simulink model "double_3D_pend"  (R2023a)
settings: Solver=VariableStepAuto  StartTime=0.0  StopTime=5  MaxStep=1e-3  RelTol=1e-9  AbsTol=1e-9  EnableMultiTasking=on
InitFcn:
  | addpath quaternion_muscle\
  | data;
values from neighbouring files (symbols this model uses):
  akt = [1,1,1]    [data.m]    (also in odvozeni_svaly.m = sym('akt',[1 6]); optim_control_nlmpc.m = u'; simulation.m = [1,1,1]*0.5)
  c = 0    [data.m]    (also in neco.m = cos(0); optim_control_nlmpc.m = 100; simulation.m = 10)
  force = [1,1,0]*(-30)    [data.m]    (also in odvozeni_svaly.m = (((length / l0m)^3) * exp(8 * length / l0m - 12.9) + (exp(-(; optim_control_nlmpc.m = [1,1,1,1,1,1]*(30); simulation.m = -[1,2,1]*1)
  g = 9.81    [data.m]    (also in optim_control_nlmpc.m; simulation.m)
  IL = [8.1667, 8.1667, 1.66667,0,0,0]    [data.m]    (also in fo_python_to_matlab.m = [ILxx ILyy ILzz ILxy ILyz ILzx]; mm_python_to_matlab.m = [ILxx ILyy ILzz ILxy ILyz ILzx]; optim_control_nlmpc.m; simulation.m = [84.1667, 84.1667, 1.66667])
  initialConditions = [1,0,0,0,0,0,zeros(1,6)]*2    [data.m]    (also in simulation.m = [1,1,1,1,1,1,0,0,0,0,0,0]*0)
  IU = [8.1667, 8.1667, 1.66667,0,0,0]    [data.m]    (also in fo_python_to_matlab.m = [IUxx IUyy IUzz IUxy IUyz IUzx]; mm_python_to_matlab.m = [IUxx IUyy IUzz IUxy IUyz IUzx]; optim_control_nlmpc.m; simulation.m = [84.1667, 84.1667, 1.66667]*1e-2)
  k = 100    [data.m]    (also in neco.m = elips_pars.k; optim_control_nlmpc.m = 0; simulation.m = 1)
  l0m = [12,25,15]    [data.m]    (also in odvozeni_svaly.m = sym('l0m', [1 6]); optim_control_nlmpc.m = [30,30,30,30,30,30]; simulation.m = [10,20,10])
  m = rand(1,2)*10    [data.m]    (also in fo_python_to_matlab.m = [m1,m2]; mm_python_to_matlab.m = [m1,m2]; neco.m = elips_pars.m; optim_control_nlmpc.m = [5,10])
  rigid1C = [0,0,5]    [data.m]    (also in fo_python_to_matlab.m = [rigid1Cx, rigid1Cy, rigid1Cz]; mm_python_to_matlab.m = [rigid1Cx, rigid1Cy, rigid1Cz]; optim_control_nlmpc.m)
  rigid1P = [0,0,-5]    [data.m]    (also in fo_python_to_matlab.m = [rigid1Px, rigid1Py, rigid1Pz]; mm_python_to_matlab.m = [rigid1Px, rigid1Py, rigid1Pz]; optim_control_nlmpc.m)
  rigid2C = [0,0,5]    [data.m]    (also in fo_python_to_matlab.m = [rigid2Cx, rigid2Cy, rigid2Cz]; mm_python_to_matlab.m = [rigid2Cx, rigid2Cy, rigid2Cz]; optim_control_nlmpc.m)
  s = sin(0)    [neco.m]
undefined symbols (not defined in the file or in its folder): Ixx, Iyy, Izz, l, q1init, q2init, X, Y, Z
libraries: sm_lib x104, nesl_utility x52
(part 5 of 5)

== matlab function double_3D_pend/MATLAB Function2 ==
  data: R output; pos1 input; vel1 input; acc1 input; pos2 input; vel2 input; acc2 input; g input
function R = fcn(pos1,vel1,acc1,pos2,vel2,acc2,g)
m1 = 5;
m2 = 10;

rigid1Cx = 0;
rigid1Cy = 0;
rigid1Cz = 5;

rigid1Px = 0;
rigid1Py = 0;
rigid1Pz = -5;

rigid2Cx = 0;
rigid2Cy = 0;
rigid2Cz = 5;

x1 = pos1(1);
x2 = pos1(2);
x3 = pos1(3);

dx1 = vel1(1);
dx2 = vel1(2);
dx3 = vel1(3);

ddx1 = acc1(1);
ddx2 = acc1(2);
ddx3 = acc1(3);

x4 = pos2(1);
x5 = pos2(2);
x6 = pos2(3);

dx4 = vel2(1);
dx5 = vel2(2);
dx6 = vel2(3);

ddx4 = acc2(1);
ddx5 = acc2(2);
ddx6 = acc2(3);

R = [m2.*((sin(x4).*sin(x6) - sin(x5).*cos(x4).*cos(x6)).*sin(x2) - (sin(x4).*sin(x5).*cos(x6) + sin(x6).*cos(x4)).*sin(x3).*cos(x2) + cos(x2).*cos(x3).*cos(x5).*cos(x6)).*(rigid2Cy.*(ddx4.*sin(x5) + ddx6 + dx4.*dx5.*cos(x5) - dx4.*(dx1.*sin(x2) + dx3).*sin(x4).*cos(x5) - dx4.*(-dx1.*sin(x3).*cos(x2) + dx2.*cos(x3)).*cos(x4).*cos(x5) - dx5.*(dx1.*sin(x2) + dx3).*sin(x5).*cos(x4) + dx5.*(-dx1.*sin(x3).*cos(x2) + dx2.*cos(x3)).*sin(x4).*sin(x5) + dx5.*(dx1.*cos(x2).*cos(x3) + dx2.*sin(x3)).*cos(x5) + (ddx1.*sin(x2) + ddx3 + dx1.*dx2.*cos(x2)).*cos(x4).*cos(x5) - (-ddx1.*sin(x3).*cos(x2) + ddx2.*cos(x3) + dx1.*dx2.*sin(x2).*sin(x3) - dx1.*dx3.*cos(x2).*cos(x3) - dx2.*dx3.*sin(x3)).*sin(x4).*cos(x5) + (ddx1.*cos(x2).*cos(x3) + ddx2.*sin(x3) - dx1.*dx2.*sin(x2).*cos(x3) - dx1.*dx3.*sin(x3).*cos(x2) + dx2.*dx3.*cos(x3)).*sin(x5)) - rigid2Cz.*(-ddx4.*sin(x6).*cos(x5) + ddx5.*cos(x6) + dx4.*dx5.*sin(x5).*sin(x6) - dx4.*dx6.*cos(x5).*cos(x6) - dx5.*dx6.*sin(x6) + dx5.*(dx1.*cos(x2).*cos(x3) + dx2.*sin(x3)).*sin(x5).*sin(x6) - dx6.*(dx1.*cos(x2).*cos(x3) + dx2.*sin(x3)).*cos(x5).*cos(x6) + (dx1.*sin(x2) + dx3).*(-dx4.*sin(x4).*sin(x5).*sin(x6) + dx4.*cos(x4).*cos(x6) + dx5.*sin(x6).*cos(x4).*cos(x5) - dx6.*sin(x4).*sin(x6) + dx6.*sin(x5).*cos(x4).*cos(x6)) + (sin(x4).*cos(x6) + sin(x5).*sin(x6).*cos(x4)).*(ddx1.*sin(x2) + ddx3 + dx1.*dx2.*cos(x2)) + (-dx1.*sin(x3).*cos(x2) + dx2.*cos(x3)).*(-dx4.*sin(x4).*cos(x6) - dx4.*sin(x5).*sin(x6).*cos(x4) - dx5.*sin(x4).*sin(x6).*cos(x5) - dx6.*sin(x4).*sin(x5).*cos(x6) - dx6.*sin(x6).*cos(x4)) + (-sin(x4).*sin(x5).*sin(x6) + cos(x4).*cos(x6)).*(-ddx1.*sin(x3).*cos(x2) + ddx2.*cos(x3) + dx1.*dx2.*sin(x2).*sin(x3) - dx1.*dx3.*cos(x2).*cos(x3) - dx2.*dx3.*sin(x3)) - (ddx1.*cos(x2).*cos(x3) + ddx2.*sin(x3) - dx1.*dx2.*sin(x2).*cos(x3) - dx1.*dx3.*sin(x3).*cos(x2) + dx2.*dx3.*cos(x3)).*sin(x6).*cos(x5)) - (-rigid2Cx.*(dx4.*sin(x5) + dx6 + (dx1.*sin(x2) + dx3).*cos(x4).*cos(x5) - (-dx1.*sin(x3).*cos(x2) + dx2.*cos(x3)).*sin(x4).*cos(x5) + (dx1.*cos(x2).*cos(x3) + dx2.*sin(x3)).*sin(x5)) + rigid2Cz.*(dx4.*cos(x5).*cos(x6) + dx5.*sin(x6) + (dx1.*sin(x2) + dx3).*(sin(x4).*sin(x6) - sin(x5).*cos(x4).*cos(x6)) + (-dx1.*sin(x3).*cos(x2) + dx2.*cos(x3)).*(sin(x4).*sin(x5).*cos(x6) + sin(x6).*cos(x4)) + (dx1.*cos(x2).*cos(x3) + dx2.*sin(x3)).*cos(x5).*cos(x6))).*(dx4.*sin(x5) + dx6 + (dx1.*sin(x2) + dx3).*cos(x4).*cos(x5) - (-dx1.*sin(x3).*cos(x2) + dx2.*cos(x3)).*sin(x4).*cos(x5) + (dx1.*cos(x2).*cos(x3) + dx2.*sin(x3)).*sin(x5)) + (rigid2Cx.*(-dx4.*sin(x6).*cos(x5) + dx5.*cos(x6) + (dx1.*sin(x2) + dx3).*(sin(x4).*cos(x6) + sin(x5).*sin(x6).*cos(x4)) + (-dx1.*sin(x3).*cos(x2) + dx2.*cos(x3)).*(-sin(x4).*sin(x5).*sin(x6) + cos(x4).*cos(x6)) - (dx1.*cos(x2).*cos(x3) + dx2.*sin(x3)).*sin(x6).*cos(x5)) - rigid2Cy.*(dx4.*cos(x5).*cos(x6) + dx5.*sin(x6) + (dx1.*sin(x2) + dx3).*(sin(x4).*sin(x6) - sin(x5).*cos(x4).*cos(x6)) + (-dx1.*sin(x3).*cos(x2) + dx2.*cos(x3)).*(sin(x4).*sin(x5).*cos(x6) + sin(x6).*cos(x4)) + (dx1.*cos(x2).*cos(x3) + dx2.*sin(x3)).*cos(x5).*cos(x6))).*(-dx4.*sin(x6).*cos(x5) + dx5.*cos(x6) + (dx1.*sin(x2) + dx3).*(sin(x4).*cos(x6) + sin(x5).*sin(x6).*cos(x4)) + (-dx1.*sin(x3).*cos(x2) + dx2.*cos(x3)).*(-sin(x4).*sin(x5).*sin(x6) + cos(x4).*cos(x6)) - (dx1.*cos(x2).*cos(x3) + dx2.*sin(x3)).*sin(x6).*cos(x5))) + m2.*((sin(x4).*cos(x6) + sin(x5).*sin(x6).*cos(x4)).*sin(x2) - (-sin(x4).*sin(x5).*sin(x6) + cos(x4).*cos(x6)).*sin(x3).*cos(x2) - sin(x6).*cos(x2).*cos(x3).*cos(x5)).*(-rigid2Cx.*(ddx4.*sin(x5) + ddx6 + dx4.*dx5.*cos(x5) - dx4.*(dx1.*sin(x2) + dx3).*sin(x4).*cos(x5) - dx4.*(-dx1.*sin(x3).*cos(x2) + dx2.*cos(x3)).*cos(x4).*cos(x5) - dx5.*(dx1.*sin(x2) + dx3).*sin(x5).*cos(x4) + dx5.*(-dx1.*sin(x3).*cos(x2) + dx2.*cos(x3)).*sin(x4).*sin(x5) + dx5.*(dx1.*cos(x2).*cos(x3) + dx2.*sin(x3)).*cos(x5) + (ddx1.*sin(x2) + ddx3 + dx1.*dx2.*cos(x2)).*cos(x4).*cos(x5) - (-ddx1.*sin(x3).*cos(x2) + ddx2.*cos(x3) + dx1.*dx2.*sin(x2).*sin(x3) - dx1.*dx3.*cos(x2).*cos(x3) - dx2.*dx3.*sin(x3)).*sin(x4).*cos(x5) + (ddx1.*cos(x2).*cos(x3) + ddx2.*sin(x3) - dx1.*dx2.*sin(x2).*cos(x3) - dx1.*dx3.*sin(x3).*cos(x2) + dx2.*dx3.*cos(x3)).*sin(x5)) + rigid2Cz.*(ddx4.*cos(x5).*cos(x6) + ddx5.*sin(x6) - dx4.*dx5.*sin(x5).*cos(x6) - dx4.*dx6.*sin(x6).*cos(x5) + dx5.*dx6.*cos(x6) - dx5.*(dx1.*cos(x2).*cos(x3) + dx2.*sin(x3)).*sin(x5).*cos(x6) - dx6.*(dx1.*cos(x2).*cos(x3) + dx2.*sin(x3)).*sin(x6).*cos(x5) + (dx1.*sin(x2) + dx3).*(dx4.*sin(x4).*sin(x5).*cos(x6) + dx4.*sin(x6).*cos(x4) - dx5.*cos(x4).*cos(x5).*cos(x6) + dx6.*sin(x4).*cos(x6) + dx6.*sin(x5).*sin(x6).*cos(x4)) + (sin(x4).*sin(x6) - sin(x5).*cos(x4).*cos(x6)).*(ddx1.*sin(x2) + ddx3 + dx1.*dx2.*cos(x2)) + (-dx1.*sin(x3).*cos(x2) + dx2.*cos(x3)).*(-dx4.*sin(x4).*sin(x6) + dx4.*sin(x5).*cos(x4).*cos(x6) + dx5.*sin(x4).*cos(x5).*cos(x6) - dx6.*sin(x4).*sin(x5).*sin(x6) + dx6.*cos(x4).*cos(x6)) + (sin(x4).*sin(x5).*cos(x6) + sin(x6).*cos(x4)).*(-ddx1.*sin(x3).*cos(x2) + ddx2.*cos(x3) + dx1.*dx2.*sin(x2).*sin(x3) - dx1.*dx3.*cos(x2).*cos(x3) - dx2.*dx3.*sin(x3)) + (ddx1.*cos(x2).*cos(x3) + ddx2.*sin(x3) - dx1.*dx2.*sin(x2).*cos(x3) - dx1.*dx3.*sin(x3).*cos(x2) + dx2.*dx3.*cos(x3)).*cos(x5).*cos(x6)) - (rigid2Cx.*(-dx4.*sin(x6).*cos(x5) + dx5.*cos(x6) + (dx1.*sin(x2) + dx3).*(sin(x4).*cos(x6) + sin(x5).*sin(x6).*cos(x4)) + (-dx1.*sin(x3).*cos(x2) + dx2.*cos(x3)).*(-sin(x4).*sin(x5).*sin(x6) + cos(x4).*cos(x6)) - (dx1.*cos(x2).*cos(x3) + dx2.*sin(x3)).*sin(x6).*cos(x5)) - rigid2Cy.*(dx4.*cos(x5).*cos(x6) + dx5.*sin(x6) + (dx1.*sin(x2) + dx3).*(sin(x4).*sin(x6) - sin(x5).*cos(x4).*cos(x6)) + (-dx1.*sin(x3).*cos(x2) + dx2.*cos(x3)).*(sin(x4).*sin(x5).*cos(x6) + sin(x6).*cos(x4)) + (dx1.*cos(x2).*cos(x3) + dx2.*sin(x3)).*cos(x5).*cos(x6))).*(dx4.*cos(x5).*cos(x6) + dx5.*sin(x6) + (dx1.*sin(x2) + dx3).*(sin(x4).*sin(x6) - sin(x5).*cos(x4).*cos(x6)) + (-dx1.*sin(x3).*cos(x2) + dx2.*cos(x3)).*(sin(x4).*sin(x5).*cos(x6) + sin(x6).*cos(x4)) + (dx1.*cos(x2).*cos(x3) + dx2.*sin(x3)).*cos(x5).*cos(x6)) + (rigid2Cy.*(dx4.*sin(x5) + dx6 + (dx1.*sin(x2) + dx3).*cos(x4).*cos(x5) - (-dx1.*sin(x3).*cos(x2) + dx2.*cos(x3)).*sin(x4).*cos(x5) + (dx1.*cos(x2).*cos(x3) + dx2.*sin(x3)).*sin(x5)) - rigid2Cz.*(-dx4.*sin(x6).*cos(x5) + dx5.*cos(x6) + (dx1.*sin(x2) + dx3).*(sin(x4).*cos(x6) + sin(x5).*sin(x6).*cos(x4)) + (-dx1.*sin(x3).*cos(x2) + dx2.*cos(x3)).*(-sin(x4).*sin(x5).*sin(x6) + cos(x4).*cos(x6)) - (dx1.*cos(x2).*cos(x3) + dx2.*sin(x3)).*sin(x6).*cos(x5))).*(dx4.*sin(x5) + dx6 + (dx1.*sin(x2) + dx3).*cos(x4).*cos(x5) - (-dx1.*sin(x3).*cos(x2) + dx2.*cos(x3)).*sin(x4).*cos(x5) + (dx1.*cos(x2).*cos(x3) + dx2.*sin(x3)).*sin(x5))) + m2.*(sin(x2).*cos(x4).*cos(x5) + sin(x3).*sin(x4).*cos(x2).*cos(x5) + sin(x5).*cos(x2).*cos(x3)).*(rigid2Cx.*(-ddx4.*sin(x6).*cos(x5) + ddx5.*cos(x6) + dx4.*dx5.*sin(x5).*sin(x6) - dx4.*dx6.*cos(x5).*cos(x6) - dx5.*dx6.*sin(x6) + dx5.*(dx1.*cos(x2).*cos(x3) + dx2.*sin(x3)).*sin(x5).*sin(x6) - dx6.*(dx1.*cos(x2).*cos(x3) + dx2.*sin(x3)).*cos(x5).*cos(x6) + (dx1.*sin(x2) + dx3).*(-dx4.*sin(x4).*sin(x5).*sin(x6) + dx4.*cos(x4).*cos(x6) + dx5.*sin(x6).*cos(x4).*cos(x5) - dx6.*sin(x4).*sin(x6) + dx6.*sin(x5).*cos(x4).*cos(x6)) + (sin(x4).*cos(x6) + sin(x5).*sin(x6).*cos(x4)).*(ddx1.*sin(x2) + ddx3 + dx1.*dx2.*cos(x2)) + (-dx1.*sin(x3).*cos(x2) + dx2.*cos(x3)).*(-dx4.*sin(x4).*cos(x6) - dx4.*sin(x5).*sin(x6).*cos(x4) - dx5.*sin(x4).*sin(x6).*cos(x5) - dx6.*sin(x4).*sin(x5).*cos(x6) - dx6.*sin(x6).*cos(x4)) + (-sin(x4).*sin(x5).*sin(x6) + cos(x4).*cos(x6)).*(-ddx1.*sin(x3).*cos(x2) + ddx2.*cos(x3) + dx1.*dx2.*sin(x2).*sin(x3) - dx1.*dx3.*cos(x2).*cos(x3) - dx2.*dx3.*sin(x3)) - (ddx1.*cos(x2).*cos(x3) + ddx2.*sin(x3) - dx1.*dx2.*sin(x2).*cos(x3) - dx1.*dx3.*sin(x3).*cos(x2) + dx2.*dx3.*cos(x3)).*sin(x6).*cos(x5)) - rigid2Cy.*(ddx4.*cos(x5).*cos(x6) + ddx5.*sin(x6) - dx4.*dx5.*sin(x5).*cos(x6) - dx4.*dx6.*sin(x6).*cos(x5) + dx5.*dx6.*cos(x6) - dx5.*(dx1.*cos(x2).*cos(x3) + dx2.*sin(x3)).*sin(x5).*cos(x6) - dx6.*(dx1.*cos(x2).*cos(x3) + dx2.*sin(x3)).*sin(x6).*cos(x5) + (dx1.*sin(x2) + dx3).*(dx4.*sin(x4).*sin(x5).*cos(x6) + dx4.*sin(x6).*cos(x4) - dx5.*cos(x4).*cos(x5).*cos(x6) + dx6.*sin(x4).*cos(x6) + dx6.*sin(x5).*sin(x6).*cos(x4)) + (sin(x4).*sin(x6) - sin(x5).*cos(x4).*cos(x6)).*(ddx1.*sin(x2) + ddx3 + dx1.*dx2.*cos(x2)) + (-dx1.*sin(x3).*cos(x2) + dx2.*cos(x3)).*(-dx4.*sin(x4).*sin(x6) + dx4.*sin(x5).*cos(x4).*cos(x6) + dx5.*sin(x4).*cos(x5).*cos(x6) - dx6.*sin(x4).*sin(x5).*sin(x6) + dx6.*cos(x4).*cos(x6)) + (sin(x4).*sin(x5).*cos(x6) + sin(x6).*cos(x4)).*(-ddx1.*sin(x3).*cos(x2) + ddx2.*cos(x3) + dx1.*dx2.*sin(x2).*sin(x3) - dx1.*dx3.*cos(x2).*cos(x3) - dx2.*dx3.*sin(x3)) + (ddx1.*cos(x2).*cos(x3) + ddx2.*sin(x3) - dx1.*dx2.*sin(x2).*cos(x3) - dx1.*dx3.*sin(x3).*cos(x2) + dx2.*dx3.*cos(x3)).*cos(x5).*cos(x6)) + (-rigid2Cx.*(dx4.*sin(x5) + dx6 + (dx1.*sin(x2) + dx3).*cos(x4).*cos(x5) - (-dx1.*sin(x3).*cos(x2) + dx2.*cos(x3)).*sin(x4).*cos(x5) + (dx1.*cos(x2).*cos(x3) + dx2.*sin(x3)).*sin(x5)) + rigid2Cz.*(dx4.*cos(x5).*cos(x6) + dx5.*sin(x6) + (dx1.*sin(x2) + dx3).*(sin(x4).*sin(x6) - sin(x5).*cos(x4).*cos(x6)) + (-dx1.*sin(x3).*cos(x2) + dx2.*cos(x3)).*(sin(x4).*sin(x5).*cos(x6) + sin(x6).*cos(x4)) + (dx1.*cos(x2).*cos(x3) + dx2.*sin(x3)).*cos(x5).*cos(x6))).*(dx4.*cos(x5).*cos(x6) + dx5.*sin(x6) + (dx1.*sin(x2) + dx3).*(sin(x4).*sin(x6) - sin(x5).*cos(x4).*cos(x6)) + (-dx1.*sin(x3).*cos(x2) + dx2.*cos(x3)).*(sin(x4).*sin(x5).*cos(x6) + sin(x6).*cos(x4)) + (dx1.*cos(x2).*cos(x3) + dx2.*sin(x3)).*cos(x5).*cos(x6)) - (rigid2Cy.*(dx4.*sin(x5) + dx6 + (dx1.*sin(x2) + dx3).*cos(x4).*cos(x5) - (-dx1.*sin(x3).*cos(x2) + dx2.*cos(x3)).*sin(x4).*cos(x5) + (dx1.*cos(x2).*cos(x3) + dx2.*sin(x3)).*sin(x5)) - rigid2Cz.*(-dx4.*sin(x6).*cos(x5) + dx5.*cos(x6) + (dx1.*sin(x2) + dx3).*(sin(x4).*cos(x6) + sin(x5).*sin(x6).*cos(x4)) + (-dx1.*sin(x3).*cos(x2) + dx2.*cos(x3)).*(-sin(x4).*sin(x5).*sin(x6) + cos(x4).*cos(x6)) - (dx1.*cos(x2).*cos(x3) + dx2.*sin(x3)).*sin(x6).*cos(x5))).*(-dx4.*sin(x6).*cos(x5) + dx5.*cos(x6) + (dx1.*sin(x2) + dx3).*(sin(x4).*cos(x6) + sin(x5).*sin(x6).*cos(x4)) + (-dx1.*sin(x3).*cos(x2) + dx2.*cos(x3)).*(-sin(x4).*sin(x5).*sin(x6) + cos(x4).*cos(x6)) - (dx1.*cos(x2).*cos(x3) + dx2.*sin(x3)).*sin(x6).*cos(x5))) - (m1.*(-rigid1Cx.*(ddx1.*sin(x2) + ddx3 + dx1.*dx2.*cos(x2)) + rigid1Cz.*(ddx1.*cos(x2).*cos(x3) + ddx2.*sin(x3) - dx1.*dx2.*sin(x2).*cos(x3) - dx1.*dx3.*sin(x3).*cos(x2) + dx2.*dx3.*cos(x3)) + (dx1.*sin(x2) + dx3).*(rigid1Cy.*(dx1.*sin(x2) + dx3) - rigid1Cz.*(-dx1.*sin(x3).*cos(x2) + dx2.*cos(x3))) - (rigid1Cx.*(-dx1.*sin(x3).*cos(x2) + dx2.*cos(x3)) - rigid1Cy.*(dx1.*cos(x2).*cos(x3) + dx2.*sin(x3))).*(dx1.*cos(x2).*cos(x3) + dx2.*sin(x3))) + m2.*(-rigid1Cx.*(ddx1.*sin(x2) + ddx3 + dx1.*dx2.*cos(x2)) + rigid1Cz.*(ddx1.*cos(x2).*cos(x3) + ddx2.*sin(x3) - dx1.*dx2.*sin(x2).*cos(x3) - dx1.*dx3.*sin(x3).*cos(x2) + dx2.*dx3.*cos(x3)) + rigid1Px.*(ddx1.*sin(x2) + ddx3 + dx1.*dx2.*cos(x2)) - rigid1Pz.*(ddx1.*cos(x2).*cos(x3) + ddx2.*sin(x3) - dx1.*dx2.*sin(x2).*cos(x3) - dx1.*dx3.*sin(x3).*cos(x2) + dx2.*dx3.*cos(x3)) + (dx1.*sin(x2) + dx3).*(rigid1Cy.*(dx1.*sin(x2) + dx3) - rigid1Cz.*(-dx1.*sin(x3).*cos(x2) + dx2.*cos(x3)) - rigid1Py.*(dx1.*sin(x2) + dx3) + rigid1Pz.*(-dx1.*sin(x3).*cos(x2) + dx2.*cos(x3))) - (dx1.*cos(x2).*cos(x3) + dx2.*sin(x3)).*(rigid1Cx.*(-dx1.*sin(x3).*cos(x2) + dx2.*cos(x3)) - rigid1Cy.*(dx1.*cos(x2).*cos(x3) + dx2.*sin(x3)) - rigid1Px.*(-dx1.*sin(x3).*cos(x2) + dx2.*cos(x3)) + rigid1Py.*(dx1.*cos(x2).*cos(x3) + dx2.*sin(x3))))).*sin(x3).*cos(x2) + (m1.*(rigid1Cx.*(-ddx1.*sin(x3).*cos(x2) + ddx2.*cos(x3) + dx1.*dx2.*sin(x2).*sin(x3) - dx1.*dx3.*cos(x2).*cos(x3) - dx2.*dx3.*sin(x3)) - rigid1Cy.*(ddx1.*cos(x2).*cos(x3) + ddx2.*sin(x3) - dx1.*dx2.*sin(x2).*cos(x3) - dx1.*dx3.*sin(x3).*cos(x2) + dx2.*dx3.*cos(x3)) + (-rigid1Cx.*(dx1.*sin(x2) + dx3) + rigid1Cz.*(dx1.*cos(x2).*cos(x3) + dx2.*sin(x3))).*(dx1.*cos(x2).*cos(x3) + dx2.*sin(x3)) - (rigid1Cy.*(dx1.*sin(x2) + dx3) - rigid1Cz.*(-dx1.*sin(x3).*cos(x2) + dx2.*cos(x3))).*(-dx1.*sin(x3).*cos(x2) + dx2.*cos(x3))) + m2.*(rigid1Cx.*(-ddx1.*sin(x3).*cos(x2) + ddx2.*cos(x3) + dx1.*dx2.*sin(x2).*sin(x3) - dx1.*dx3.*cos(x2).*cos(x3) - dx2.*dx3.*sin(x3)) - rigid1Cy.*(ddx1.*cos(x2).*cos(x3) + ddx2.*sin(x3) - dx1.*dx2.*sin(x2).*cos(x3) - dx1.*dx3.*sin(x3).*cos(x2) + dx2.*dx3.*cos(x3)) - rigid1Px.*(-ddx1.*sin(x3).*cos(x2) + ddx2.*cos(x3) + dx1.*dx2.*sin(x2).*sin(x3) - dx1.*dx3.*cos(x2).*cos(x3) - dx2.*dx3.*sin(x3)) + rigid1Py.*(ddx1.*cos(x2).*cos(x3) + ddx2.*sin(x3) - dx1.*dx2.*sin(x2).*cos(x3) - dx1.*dx3.*sin(x3).*cos(x2) + dx2.*dx3.*cos(x3)) - (-dx1.*sin(x3).*cos(x2) + dx2.*cos(x3)).*(rigid1Cy.*(dx1.*sin(x2) + dx3) - rigid1Cz.*(-dx1.*sin(x3).*cos(x2) + dx2.*cos(x3)) - rigid1Py.*(dx1.*sin(x2) + dx3) + rigid1Pz.*(-dx1.*sin(x3).*cos(x2) + dx2.*cos(x3))) + (dx1.*cos(x2).*cos(x3) + dx2.*sin(x3)).*(-rigid1Cx.*(dx1.*sin(x2) + dx3) + rigid1Cz.*(dx1.*cos(x2).*cos(x3) + dx2.*sin(x3)) + rigid1Px.*(dx1.*sin(x2) + dx3) - rigid1Pz.*(dx1.*cos(x2).*cos(x3) + dx2.*sin(x3))))).*sin(x2) + (m1.*(rigid1Cy.*(ddx1.*sin(x2) + ddx3 + dx1.*dx2.*cos(x2)) - rigid1Cz.*(-ddx1.*sin(x3).*cos(x2) + ddx2.*cos(x3) + dx1.*dx2.*sin(x2).*sin(x3) - dx1.*dx3.*cos(x2).*cos(x3) - dx2.*dx3.*sin(x3)) - (dx1.*sin(x2) + dx3).*(-rigid1Cx.*(dx1.*sin(x2) + dx3) + rigid1Cz.*(dx1.*cos(x2).*cos(x3) + dx2.*sin(x3))) + (rigid1Cx.*(-dx1.*sin(x3).*cos(x2) + dx2.*cos(x3)) - rigid1Cy.*(dx1.*cos(x2).*cos(x3) + dx2.*sin(x3))).*(-dx1.*sin(x3).*cos(x2) + dx2.*cos(x3))) + m2.*(rigid1Cy.*(ddx1.*sin(x2) + ddx3 + dx1.*dx2.*cos(x2)) - rigid1Cz.*(-ddx1.*sin(x3).*cos(x2) + ddx2.*cos(x3) + dx1.*dx2.*sin(x2).*sin(x3) - dx1.*dx3.*cos(x2).*cos(x3) - dx2.*dx3.*sin(x3)) - rigid1Py.*(ddx1.*sin(x2) + ddx3 + dx1.*dx2.*cos(x2)) + rigid1Pz.*(-ddx1.*sin(x3).*cos(x2) + ddx2.*cos(x3) + dx1.*dx2.*sin(x2).*sin(x3) - dx1.*dx3.*cos(x2).*cos(x3) - dx2.*dx3.*sin(x3)) - (dx1.*sin(x2) + dx3).*(-rigid1Cx.*(dx1.*sin(x2) + dx3) + rigid1Cz.*(dx1.*cos(x2).*cos(x3) + dx2.*sin(x3)) + rigid1Px.*(dx1.*sin(x2) + dx3) - rigid1Pz.*(dx1.*cos(x2).*cos(x3) + dx2.*sin(x3))) + (-dx1.*sin(x3).*cos(x2) + dx2.*cos(x3)).*(rigid1Cx.*(-dx1.*sin(x3).*cos(x2) + dx2.*cos(x3)) - rigid1Cy.*(dx1.*cos(x2).*cos(x3) + dx2.*sin(x3)) - rigid1Px.*(-dx1.*sin(x3).*cos(x2) + dx2.*cos(x3)) + rigid1Py.*(dx1.*cos(x2).*cos(x3) + dx2.*sin(x3))))).*cos(x2).*cos(x3); m2.*(-(sin(x4).*sin(x6) - sin(x5).*cos(x4).*cos(x6)).*sin(x1).*cos(x2) + (-sin(x1).*sin(x2).*sin(x3) + cos(x1).*cos(x3)).*(sin(x4).*sin(x5).*cos(x6) + sin(x6).*cos(x4)) + (sin(x1).*sin(x2).*cos(x3) + sin(x3).*cos(x1)).*cos(x5).*cos(x6)).*(rigid2Cy.*(ddx4.*sin(x5) + ddx6 + dx4.*dx5.*cos(x5) - dx4.*(dx1.*sin(x2) + dx3).*sin(x4).*cos(x5) - dx4.*(-dx1.*sin(x3).*cos(x2) + dx2.*cos(x3)).*cos(x4).*cos(x5) - dx5.*(dx1.*sin(x2) + dx3).*sin(x5).*cos(x4) + dx5.*(-dx1.*sin(x3).*cos(x2) + dx2.*cos(x3)).*sin(x4).*sin(x5) + dx5.*(dx1.*cos(x2).*cos(x3) + dx2.*sin(x3)).*cos(x5) + (ddx1.*sin(x2) + ddx3 + dx1.*dx2.*cos(x2)).*cos(x4).*cos(x5) - (-ddx1.*sin(x3).*cos(x2) + ddx2.*cos(x3) + dx1.*dx2.*sin(x2).*sin(x3) - dx1.*dx3.*cos(x2).*cos(x3) - dx2.*dx3.*sin(x3)).*sin(x4).*cos(x5) + (ddx1.*cos(x2).*cos(x3) + ddx2.*sin(x3) - dx1.*dx2.*sin(x2).*cos(x3) - dx1.*dx3.*sin(x3).*cos(x2) + dx2.*dx3.*cos(x3)).*sin(x5)) - rigid2Cz.*(-ddx4.*sin(x6).*cos(x5) + ddx5.*cos(x6) + dx4.*dx5.*sin(x5).*sin(x6) - dx4.*dx6.*cos(x5).*cos(x6) - dx5.*dx6.*sin(x6) + dx5.*(dx1.*cos(x2).*cos(x3) + dx2.*sin(x3)).*sin(x5).*sin(x6) - dx6.*(dx1.*cos(x2).*cos(x3) + dx2.*sin(x3)).*cos(x5).*cos(x6) + (dx1.*sin(x2) + dx3).*(-dx4.*sin(x4).*sin(x5).*sin(x6) + dx4.*cos(x4).*cos(x6) + dx5.*sin(x6).*cos(x4).*cos(x5) - dx6.*sin(x4).*sin(x6) + dx6.*sin(x5).*cos(x4).*cos(x6)) + (sin(x4).*cos(x6) + sin(x5).*sin(x6).*cos(x4)).*(ddx1.*sin(x2) + ddx3 + dx1.*dx2.*cos(x2)) + (-dx1.*sin(x3).*cos(x2) + dx2.*cos(x3)).*(-dx4.*sin(x4).*cos(x6) - dx4.*sin(x5).*sin(x6).*cos(x4) - dx5.*sin(x4).*sin(x6).*cos(x5) - dx6.*sin(x4).*sin(x5).*cos(x6) - dx6.*sin(x6).*cos(x4)) + (-sin(x4).*sin(x5).*sin(x6) + cos(x4).*cos(x6)).*(-ddx1.*sin(x3).*cos(x2) + ddx2.*cos(x3) + dx1.*dx2.*sin(x2).*sin(x3) - dx1.*dx3.*cos(x2).*cos(x3) - dx2.*dx3.*sin(x3)) - (ddx1.*cos(x2).*cos(x3) + ddx2.*sin(x3) - dx1.*dx2.*sin(x2).*cos(x3) - dx1.*dx3.*sin(x3).*cos(x2) + dx2.*dx3.*cos(x3)).*sin(x6).*cos(x5)) - (-rigid2Cx.*(dx4.*sin(x5) + dx6 + (dx1.*sin(x2) + dx3).*cos(x4).*cos(x5) - (-dx1.*sin(x3).*cos(x2) + dx2.*cos(x3)).*sin(x4).*cos(x5) + (dx1.*cos(x2).*cos(x3) + dx2.*sin(x3)).*sin(x5)) + rigid2Cz.*(dx4.*cos(x5).*cos(x6) + dx5.*sin(x6) + (dx1.*sin(x2) + dx3).*(sin(x4).*sin(x6) - sin(x5).*cos(x4).*cos(x6)) + (-dx1.*sin(x3).*cos(x2) + dx2.*cos(x3)).*(sin(x4).*sin(x5).*cos(x6) + sin(x6).*cos(x4)) + (dx1.*cos(x2).*cos(x3) + dx2.*sin(x3)).*cos(x5).*cos(x6))).*(dx4.*sin(x5) + dx6 + (dx1.*sin(x2) + dx3).*cos(x4).*cos(x5) - (-dx1.*sin(x3).*cos(x2) + dx2.*cos(x3)).*sin(x4).*cos(x5) + (dx1.*cos(x2).*cos(x3) + dx2.*sin(x3)).*sin(x5)) + (rigid2Cx.*(-dx4.*sin(x6).*cos(x5) + dx5.*cos(x6) + (dx1.*sin(x2) + dx3).*(sin(x4).*cos(x6) + sin(x5).*sin(x6).*cos(x4)) + (-dx1.*sin(x3).*cos(x2) + dx2.*cos(x3)).*(-sin(x4).*sin(x5).*sin(x6) + cos(x4).*cos(x6)) - (dx1.*cos(x2).*cos(x3) + dx2.*sin(x3)).*sin(x6).*cos(x5)) - rigid2Cy.*(dx4.*cos(x5).*cos(x6) + dx5.*sin(x6) + (dx1.*sin(x2) + dx3).*(sin(x4).*sin(x6) - sin(x5).*cos(x4).*cos(x6)) + (-dx1.*sin(x3).*cos(x2) + dx2.*cos(x3)).*(sin(x4).*sin(x5).*cos(x6) + sin(x6).*cos(x4)) + (dx1.*cos(x2).*cos(x3) + dx2.*sin(x3)).*cos(x5).*cos(x6))).*(-dx4.*sin(x6).*cos(x5) + dx5.*cos(x6) + (dx1.*sin(x2) + dx3).*(sin(x4).*cos(x6) + sin(x5).*sin(x6).*cos(x4)) + (-dx1.*sin(x3).*cos(x2) + dx2.*cos(x3)).*(-sin(x4).*sin(x5).*sin(x6) + cos(x4).*cos(x6)) - (dx1.*cos(x2).*cos(x3) + dx2.*sin(x3)).*sin(x6).*cos(x5))) + m2.*(-(sin(x4).*cos(x6) + sin(x5).*sin(x6).*cos(x4)).*sin(x1).*cos(x2) + (-sin(x1).*sin(x2).*sin(x3) + cos(x1).*cos(x3)).*(-sin(x4).*sin(x5).*sin(x6) + cos(x4).*cos(x6)) - (sin(x1).*sin(x2).*cos(x3) + sin(x3).*cos(x1)).*sin(x6).*cos(x5)).*(-rigid2Cx.*(ddx4.*sin(x5) + ddx6 + dx4.*dx5.*cos(x5) - dx4.*(dx1.*sin(x2) + dx3).*sin(x4).*cos(x5) - dx4.*(-dx1.*sin(x3).*cos(x2) + dx2.*cos(x3)).*cos(x4).*cos(x5) - dx5.*(dx1.*sin(x2) + dx3).*sin(x5).*cos(x4) + dx5.*(-dx1.*sin(x3).*cos(x2) + dx2.*cos(x3)).*sin(x4).*sin(x5) + dx5.*(dx1.*cos(x2).*cos(x3) + dx2.*sin(x3)).*cos(x5) + (ddx1.*sin(x2) + ddx3 + dx1.*dx2.*cos(x2)).*cos(x4).*cos(x5) - (-ddx1.*sin(x3).*cos(x2) + ddx2.*cos(x3) + dx1.*dx2.*sin(x2).*sin(x3) - dx1.*dx3.*cos(x2).*cos(x3) - dx2.*dx3.*sin(x3)).*sin(x4).*cos(x5) + (ddx1.*cos(x2).*cos(x3) + ddx2.*sin(x3) - dx1.*dx2.*sin(x2).*cos(x3) - dx1.*dx3.*sin(x3).*cos(x2) + dx2.*dx3.*cos(x3)).*sin(x5)) + rigid2Cz.*(ddx4.*cos(x5).*cos(x6) + ddx5.*sin(x6) - dx4.*dx5.*sin(x5).*cos(x6) - dx4.*dx6.*sin(x6).*cos(x5) + dx5.*dx6.*cos(x6) - dx5.*(dx1.*cos(x2).*cos(x3) + dx2.*sin(x3)).*sin(x5).*cos(x6) - dx6.*(dx1.*cos(x2).*cos(x3) + dx2.*sin(x3)).*sin(x6).*cos(x5) + (dx1.*sin(x2) + dx3).*(dx4.*sin(x4).*sin(x5).*cos(x6) + dx4.*sin(x6).*cos(x4) - dx5.*cos(x4).*cos(x5).*cos(x6) + dx6.*sin(x4).*cos(x6) + dx6.*sin(x5).*sin(x6).*cos(x4)) + (sin(x4).*sin(x6) - sin(x5).*cos(x4).*cos(x6)).*(ddx1.*sin(x2) + ddx3 + dx1.*dx2.*cos(x2)) + (-dx1.*sin(x3).*cos(x2) + dx2.*cos(x3)).*(-dx4.*sin(x4).*sin(x6) + dx4.*sin(x5).*cos(x4).*cos(x6) + dx5.*sin(x4).*cos(x5).*cos(x6) - dx6.*sin(x4).*sin(x5).*sin(x6) + dx6.*cos(x4).*cos(x6)) + (sin(x4).*sin(x5).*cos(x6) + sin(x6).*cos(x4)).*(-ddx1.*sin(x3).*cos(x2) + ddx2.*cos(x3) + dx1.*dx2.*sin(x2).*sin(x3) - dx1.*dx3.*cos(x2).*cos(x3) - dx2.*dx3.*sin(x3)) + (ddx1.*cos(x2).*cos(x3) + ddx2.*sin(x3) - dx1.*dx2.*sin(x2).*cos(x3) - dx1.*dx3.*sin(x3).*cos(x2) + dx2.*dx3.*cos(x3)).*cos(x5).*cos(x6)) - (rigid2Cx.*(-dx4.*sin(x6).*cos(x5) + dx5.*cos(x6) + (dx1.*sin(x2) + dx3).*(sin(x4).*cos(x6) + sin(x5).*sin(x6).*cos(x4)) + (-dx1.*sin(x3).*cos(x2) + dx2.*cos(x3)).*(-sin(x4).*sin(x5).*sin(x6) + cos(x4).*cos(x6)) - (dx1.*cos(x2).*cos(x3) + dx2.*sin(x3)).*sin(x6).*cos(x5)) - rigid2Cy.*(dx4.*cos(x5).*cos(x6) + dx5.*sin(x6) + (dx1.*sin(x2) + dx3).*(sin(x4).*sin(x6) - sin(x5).*cos(x4).*cos(x6)) + (-dx1.*sin(x3).*cos(x2) + dx2.*cos(x3)).*(sin(x4).*sin(x5).*cos(x6) + sin(x6).*cos(x4)) + (dx1.*cos(x2).*cos(x3) + dx2.*sin(x3)).*cos(x5).*cos(x6))).*(dx4.*cos(x5).*cos(x6) + dx5.*sin(x6) + (dx1.*sin(x2) + dx3).*(sin(x4).*sin(x6) - sin(x5).*cos(x4).*cos(x6)) + (-dx1.*sin(x3).*cos(x2) + dx2.*cos(x3)).*(sin(x4).*sin(x5).*cos(x6) + sin(x6).*cos(x4)) + (dx1.*cos(x2).*cos(x3) + dx2.*sin(x3)).*cos(x5).*cos(x6)) + (rigid2Cy.*(dx4.*sin(x5) + dx6 + (dx1.*sin(x2) + dx3).*cos(x4).*cos(x5) - (-dx1.*sin(x3).*cos(x2) + dx2.*cos(x3)).*sin(x4).*cos(x5) + (dx1.*cos(x2).*cos(x3) + dx2.*sin(x3)).*sin(x5)) - rigid2Cz.*(-dx4.*sin(x6).*cos(x5) + dx5.*cos(x6) + (dx1.*sin(x2) + dx3).*(sin(x4).*cos(x6) + sin(x5).*sin(x6).*cos(x4)) + (-dx1.*sin(x3).*cos(x2) + dx2.*cos(x3)).*(-sin(x4).*sin(x5).*sin(x6) + cos(x4).*cos(x6)) - (dx1.*cos(x2).*cos(x3) + dx2.*sin(x3)).*sin(x6).*cos(x5))).*(dx4.*sin(x5) + dx6 + (dx1.*sin(x2) + dx3).*cos(x4).*cos(x5) - (-dx1.*sin(x3).*cos(x2) + dx2.*cos(x3)).*sin(x4).*cos(x5) + (dx1.*cos(x2).*cos(x3) + dx2.*sin(x3)).*sin(x5))) + m2.*(-(-sin(x1).*sin(x2).*sin(x3) + cos(x1).*cos(x3)).*sin(x4).*cos(x5) + (sin(x1).*sin(x2).*cos(x3) + sin(x3).*cos(x1)).*sin(x5) - sin(x1).*cos(x2).*cos(x4).*cos(x5)).*(rigid2Cx.*(-ddx4.*sin(x6).*cos(x5) + ddx5.*cos(x6) + dx4.*dx5.*sin(x5).*sin(x6) - dx4.*dx6.*cos(x5).*cos(x6) - dx5.*dx6.*sin(x6) + dx5.*(dx1.*cos(x2).*cos(x3) + dx2.*sin(x3)).*sin(x5).*sin(x6) - dx6.*(dx1.*cos(x2).*cos(x3) + dx2.*sin(x3)).*cos(x5).*cos(x6) + (dx1.*sin(x2) + dx3).*(-dx4.*sin(x4).*sin(x5).*sin(x6) + dx4.*cos(x4).*cos(x6) + dx5.*sin(x6).*cos(x4).*cos(x5) - dx6.*sin(x4).*sin(x6) + dx6.*sin(x5).*cos(x4).*cos(x6)) + (sin(x4).*cos(x6) + sin(x5).*sin(x6).*cos(x4)).*(ddx1.*sin(x2) + ddx3 + dx1.*dx2.*cos(x2)) + (-dx1.*sin(x3).*cos(x2) + dx2.*cos(x3)).*(-dx4.*sin(x4).*cos(x6) - dx4.*sin(x5).*sin(x6).*cos(x4) - dx5.*sin(x4).*sin(x6).*cos(x5) - dx6.*sin(x4).*sin(x5).*cos(x6) - dx6.*sin(x6).*cos(x4)) + (-sin(x4).*sin(x5).*sin(x6) + cos(x4).*cos(x6)).*(-ddx1.*sin(x3).*cos(x2) + ddx2.*cos(x3) + dx1.*dx2.*sin(x2).*sin(x3) - dx1.*dx3.*cos(x2).*cos(x3) - dx2.*dx3.*sin(x3)) - (ddx1.*cos(x2).*cos(x3) + ddx2.*sin(x3) - dx1.*dx2.*sin(x2).*cos(x3) - dx1.*dx3.*sin(x3).*cos(x2) + dx2.*dx3.*cos(x3)).*sin(x6).*cos(x5)) - rigid2Cy.*(ddx4.*cos(x5).*cos(x6) + ddx5.*sin(x6) - dx4.*dx5.*sin(x5).*cos(x6) - dx4.*dx6.*sin(x6).*cos(x5) + dx5.*dx6.*cos(x6) - dx5.*(dx1.*cos(x2).*cos(x3) + dx2.*sin(x3)).*sin(x5).*cos(x6) - dx6.*(dx1.*cos(x2).*cos(x3) + dx2.*sin(x3)).*sin(x6).*cos(x5) + (dx1.*sin(x2) + dx3).*(dx4.*sin(x4).*sin(x5).*cos(x6) + dx4.*sin(x6).*cos(x4) - dx5.*cos(x4).*cos(x5).*cos(x6) + dx6.*sin(x4).*cos(x6) + dx6.*sin(x5).*sin(x6).*cos(x4)) + (sin(x4).*sin(x6) - sin(x5).*cos(x4).*cos(x6)).*(ddx1.*sin(x2) + ddx3 + dx1.*dx2.*cos(x2)) + (-dx1.*sin(x3).*cos(x2) + dx2.*cos(x3)).*(-dx4.*sin(x4).*sin(x6) + dx4.*sin(x5).*cos(x4).*cos(x6) + dx5.*sin(x4).*cos(x5).*cos(x6) - dx6.*sin(x4).*sin(x5).*sin(x6) + dx6.*cos(x4).*cos(x6)) + (sin(x4).*sin(x5).*cos(x6) + sin(x6).*cos(x4)).*(-ddx1.*sin(x3).*cos(x2) + ddx2.*cos(x3) + dx1.*dx2.*sin(x2).*sin(x3) - dx1.*dx3.*cos(x2).*cos(x3) - dx2.*dx3.*sin(x3)) + (ddx1.*cos(x2).*cos(x3) + ddx2.*sin(x3) - dx1.*dx2.*sin(x2).*cos(x3) - dx1.*dx3.*sin(x3).*cos(x2) + dx2.*dx3.*cos(x3)).*cos(x5).*cos(x6)) + (-rigid2Cx.*(dx4.*sin(x5) + dx6 + (dx1.*sin(x2) + dx3).*cos(x4).*cos(x5) - (-dx1.*sin(x3).*cos(x2) + dx2.*cos(x3)).*sin(x4).*cos(x5) + (dx1.*cos(x2).*cos(x3) + dx2.*sin(x3)).*sin(x5)) + rigid2Cz.*(dx4.*cos(x5).*cos(x6) + dx5.*sin(x6) + (dx1.*sin(x2) + dx3).*(sin(x4).*sin(x6) - sin(x5).*cos(x4).*cos(x6)) + (-dx1.*sin(x3).*cos(x2) + dx2.*cos(x3)).*(sin(x4).*sin(x5).*cos(x6) + sin(x6).*cos(x4)) + (dx1.*cos(x2).*cos(x3) + dx2.*sin(x3)).*cos(x5).*cos(x6))).*(dx4.*cos(x5).*cos(x6) + dx5.*sin(x6) + (dx1.*sin(x2) + dx3).*(sin(x4).*sin(x6) - sin(x5).*cos(x4).*cos(x6)) + (-dx1.*sin(x3).*cos(x2) + dx2.*cos(x3)).*(sin(x4).*sin(x5).*cos(x6) + sin(x6).*cos(x4)) + (dx1.*cos(x2).*cos(x3) + dx2.*sin(x3)).*cos(x5).*cos(x6)) - (rigid2Cy.*(dx4.*sin(x5) + dx6 + (dx1.*sin(x2) + dx3).*cos(x4).*cos(x5) - (-dx1.*sin(x3).*cos(x2) + dx2.*cos(x3)).*sin(x4).*cos(x5) + (dx1.*cos(x2).*cos(x3) + dx2.*sin(x3)).*sin(x5)) - rigid2Cz.*(-dx4.*sin(x6).*cos(x5) + dx5.*cos(x6) + (dx1.*sin(x2) + dx3).*(sin(x4).*cos(x6) + sin(x5).*sin(x6).*cos(x4)) + (-dx1.*sin(x3).*cos(x2) + dx2.*cos(x3)).*(-sin(x4).*sin(x5).*sin(x6) + cos(x4).*cos(x6)) - (dx1.*cos(x2).*cos(x3) + dx2.*sin(x3)).*sin(x6).*cos(x5))).*(-dx4.*sin(x6).*cos(x5) + dx5.*cos(x6) + (dx1.*sin(x2) + dx3).*(sin(x4).*cos(x6) + sin(x5).*sin(x6).*cos(x4)) + (-dx1.*sin(x3).*cos(x2) + dx2.*cos(x3)).*(-sin(x4).*sin(x5).*sin(x6) + cos(x4).*cos(x6)) - (dx1.*cos(x2).*cos(x3) + dx2.*sin(x3)).*sin(x6).*cos(x5))) + (m1.*(-rigid1Cx.*(ddx1.*sin(x2) + ddx3 + dx1.*dx2.*cos(x2)) + rigid1Cz.*(ddx1.*cos(x2).*cos(x3) + ddx2.*sin(x3) - dx1.*dx2.*sin(x2).*cos(x3) - dx1.*dx3.*sin(x3).*cos(x2) + dx2.*dx3.*cos(x3)) + (dx1.*sin(x2) + dx3).*(rigid1Cy.*(dx1.*sin(x2) + dx3) - rigid1Cz.*(-dx1.*sin(x3).*cos(x2) + dx2.*cos(x3))) - (rigid1Cx.*(-dx1.*sin(x3).*cos(x2) + dx2.*cos(x3)) - rigid1Cy.*(dx1.*cos(x2).*cos(x3) + dx2.*sin(x3))).*(dx1.*cos(x2).*cos(x3) + dx2.*sin(x3))) + m2.*(-rigid1Cx.*(ddx1.*sin(x2) + ddx3 + dx1.*dx2.*cos(x2)) + rigid1Cz.*(ddx1.*cos(x2).*cos(x3) + ddx2.*sin(x3) - dx1.*dx2.*sin(x2).*cos(x3) - dx1.*dx3.*sin(x3).*cos(x2) + dx2.*dx3.*cos(x3)) + rigid1Px.*(ddx1.*sin(x2) + ddx3 + dx1.*dx2.*cos(x2)) - rigid1Pz.*(ddx1.*cos(x2).*cos(x3) + ddx2.*sin(x3) - dx1.*dx2.*sin(x2).*cos(x3) - dx1.*dx3.*sin(x3).*cos(x2) + dx2.*dx3.*cos(x3)) + (dx1.*sin(x2) + dx3).*(rigid1Cy.*(dx1.*sin(x2) + dx3) - rigid1Cz.*(-dx1.*sin(x3).*cos(x2) + dx2.*cos(x3)) - rigid1Py.*(dx1.*sin(x2) + dx3) + rigid1Pz.*(-dx1.*sin(x3).*cos(x2) + dx2.*cos(x3))) - (dx1.*cos(x2).*cos(x3) + dx2.*sin(x3)).*(rigid1Cx.*(-dx1.*sin(x3).*cos(x2) + dx2.*cos(x3)) - rigid1Cy.*(dx1.*cos(x2).*cos(x3) + dx2.*sin(x3)) - rigid1Px.*(-dx1.*sin(x3).*cos(x2) + dx2.*cos(x3)) + rigid1Py.*(dx1.*cos(x2).*cos(x3) + dx2.*sin(x3))))).*(-sin(x1).*sin(x2).*sin(x3) + cos(x1).*cos(x3)) - (m1.*(rigid1Cx.*(-ddx1.*sin(x3).*cos(x2) + ddx2.*cos(x3) + dx1.*dx2.*sin(x2).*sin(x3) - dx1.*dx3.*cos(x2).*cos(x3) - dx2.*dx3.*sin(x3)) - rigid1Cy.*(ddx1.*cos(x2).*cos(x3) + ddx2.*sin(x3) - dx1.*dx2.*sin(x2).*cos(x3) - dx1.*dx3.*sin(x3).*cos(x2) + dx2.*dx3.*cos(x3)) + (-rigid1Cx.*(dx1.*sin(x2) + dx3) + rigid1Cz.*(dx1.*cos(x2).*cos(x3) + dx2.*sin(x3))).*(dx1.*cos(x2).*cos(x3) + dx2.*sin(x3)) - (rigid1Cy.*(dx1.*sin(x2) + dx3) - rigid1Cz.*(-dx1.*sin(x3).*cos(x2) + dx2.*cos(x3))).*(-dx1.*sin(x3).*cos(x2) + dx2.*cos(x3))) + m2.*(rigid1Cx.*(-ddx1.*sin(x3).*cos(x2) + ddx2.*cos(x3) + dx1.*dx2.*sin(x2).*sin(x3) - dx1.*dx3.*cos(x2).*cos(x3) - dx2.*dx3.*sin(x3)) - rigid1Cy.*(ddx1.*cos(x2).*cos(x3) + ddx2.*sin(x3) - dx1.*dx2.*sin(x2).*cos(x3) - dx1.*dx3.*sin(x3).*cos(x2) + dx2.*dx3.*cos(x3)) - rigid1Px.*(-ddx1.*sin(x3).*cos(x2) + ddx2.*cos(x3) + dx1.*dx2.*sin(x2).*sin(x3) - dx1.*dx3.*cos(x2).*cos(x3) - dx2.*dx3.*sin(x3)) + rigid1Py.*(ddx1.*cos(x2).*cos(x3) + ddx2.*sin(x3) - dx1.*dx2.*sin(x2).*cos(x3) - dx1.*dx3.*sin(x3).*cos(x2) + dx2.*dx3.*cos(x3)) - (-dx1.*sin(x3).*cos(x2) + dx2.*cos(x3)).*(rigid1Cy.*(dx1.*sin(x2) + dx3) - rigid1Cz.*(-dx1.*sin(x3).*cos(x2) + dx2.*cos(x3)) - rigid1Py.*(dx1.*sin(x2) + dx3) + rigid1Pz.*(-dx1.*sin(x3).*cos(x2) + dx2.*cos(x3))) + (dx1.*cos(x2).*cos(x3) + dx2.*sin(x3)).*(-rigid1Cx.*(dx1.*sin(x2) + dx3) + rigid1Cz.*(dx1.*cos(x2).*cos(x3) + dx2.*sin(x3)) + rigid1Px.*(dx1.*sin(x2) + dx3) - rigid1Pz.*(dx1.*cos(x2).*cos(x3) + dx2.*sin(x3))))).*sin(x1).*cos(x2) + (m1.*(rigid1Cy.*(ddx1.*sin(x2) + ddx3 + dx1.*dx2.*cos(x2)) - rigid1Cz.*(-ddx1.*sin(x3).*cos(x2) + ddx2.*cos(x3) + dx1.*dx2.*sin(x2).*sin(x3) - dx1.*dx3.*cos(x2).*cos(x3) - dx2.*dx3.*sin(x3)) - (dx1.*sin(x2) + dx3).*(-rigid1Cx.*(dx1.*sin(x2) + dx3) + rigid1Cz.*(dx1.*cos(x2).*cos(x3) + dx2.*sin(x3))) + (rigid1Cx.*(-dx1.*sin(x3).*cos(x2) + dx2.*cos(x3)) - rigid1Cy.*(dx1.*cos(x2).*cos(x3) + dx2.*sin(x3))).*(-dx1.*sin(x3).*cos(x2) + dx2.*cos(x3))) + m2.*(rigid1Cy.*(ddx1.*sin(x2) + ddx3 + dx1.*dx2.*cos(x2)) - rigid1Cz.*(-ddx1.*sin(x3).*cos(x2) + ddx2.*cos(x3) + dx1.*dx2.*sin(x2).*sin(x3) - dx1.*dx3.*cos(x2).*cos(x3) - dx2.*dx3.*sin(x3)) - rigid1Py.*(ddx1.*sin(x2) + ddx3 + dx1.*dx2.*cos(x2)) + rigid1Pz.*(-ddx1.*sin(x3).*cos(x2) + ddx2.*cos(x3) + dx1.*dx2.*sin(x2).*sin(x3) - dx1.*dx3.*cos(x2).*cos(x3) - dx2.*dx3.*sin(x3)) - (dx1.*sin(x2) + dx3).*(-rigid1Cx.*(dx1.*sin(x2) + dx3) + rigid1Cz.*(dx1.*cos(x2).*cos(x3) + dx2.*sin(x3)) + rigid1Px.*(dx1.*sin(x2) + dx3) - rigid1Pz.*(dx1.*cos(x2).*cos(x3) + dx2.*sin(x3))) + (-dx1.*sin(x3).*cos(x2) + dx2.*cos(x3)).*(rigid1Cx.*(-dx1.*sin(x3).*cos(x2) + dx2.*cos(x3)) - rigid1Cy.*(dx1.*cos(x2).*cos(x3) + dx2.*sin(x3)) - rigid1Px.*(-dx1.*sin(x3).*cos(x2) + dx2.*cos(x3)) + rigid1Py.*(dx1.*cos(x2).*cos(x3) + dx2.*sin(x3))))).*(sin(x1).*sin(x2).*cos(x3) + sin(x3).*cos(x1)); g.*m1 + g.*m2 + m2.*((sin(x1).*sin(x3) - sin(x2).*cos(x1).*cos(x3)).*sin(x5) - (sin(x1).*cos(x3) + sin(x2).*sin(x3).*cos(x1)).*sin(x4).*cos(x5) + cos(x1).*cos(x2).*cos(x4).*cos(x5)).*(rigid2Cx.*(-ddx4.*sin(x6).*cos(x5) + ddx5.*cos(x6) + dx4.*dx5.*sin(x5).*sin(x6) - dx4.*dx6.*cos(x5).*cos(x6) - dx5.*dx6.*sin(x6) + dx5.*(dx1.*cos(x2).*cos(x3) + dx2.*sin(x3)).*sin(x5).*sin(x6) - dx6.*(dx1.*cos(x2).*cos(x3) + dx2.*sin(x3)).*cos(x5).*cos(x6) + (dx1.*sin(x2) + dx3).*(-dx4.*sin(x4).*sin(x5).*sin(x6) + dx4.*cos(x4).*cos(x6) + dx5.*sin(x6).*cos(x4).*cos(x5) - dx6.*sin(x4).*sin(x6) + dx6.*sin(x5).*cos(x4).*cos(x6)) + (sin(x4).*cos(x6) + sin(x5).*sin(x6).*cos(x4)).*(ddx1.*sin(x2) + ddx3 + dx1.*dx2.*cos(x2)) + (-dx1.*sin(x3).*cos(x2) + dx2.*cos(x3)).*(-dx4.*sin(x4).*cos(x6) - dx4.*sin(x5).*sin(x6).*cos(x4) - dx5.*sin(x4).*sin(x6).*cos(x5) - dx6.*sin(x4).*sin(x5).*cos(x6) - dx6.*sin(x6).*cos(x4)) + (-sin(x4).*sin(x5).*sin(x6) + cos(x4).*cos(x6)).*(-ddx1.*sin(x3).*cos(x2) + ddx2.*cos(x3) + dx1.*dx2.*sin(x2).*sin(x3) - dx1.*dx3.*cos(x2).*cos(x3) - dx2.*dx3.*sin(x3)) - (ddx1.*cos(x2).*cos(x3) + ddx2.*sin(x3) - dx1.*dx2.*sin(x2).*cos(x3) - dx1.*dx3.*sin(x3).*cos(x2) + dx2.*dx3.*cos(x3)).*sin(x6).*cos(x5)) - rigid2Cy.*(ddx4.*cos(x5).*cos(x6) + ddx5.*sin(x6) - dx4.*dx5.*sin(x5).*cos(x6) - dx4.*dx6.*sin(x6).*cos(x5) + dx5.*dx6.*cos(x6) - dx5.*(dx1.*cos(x2).*cos(x3) + dx2.*sin(x3)).*sin(x5).*cos(x6) - dx6.*(dx1.*cos(x2).*cos(x3) + dx2.*sin(x3)).*sin(x6).*cos(x5) + (dx1.*sin(x2) + dx3).*(dx4.*sin(x4).*sin(x5).*cos(x6) + dx4.*sin(x6).*cos(x4) - dx5.*cos(x4).*cos(x5).*cos(x6) + dx6.*sin(x4).*cos(x6) + dx6.*sin(x5).*sin(x6).*cos(x4)) + (sin(x4).*sin(x6) - sin(x5).*cos(x4).*cos(x6)).*(ddx1.*sin(x2) + ddx3 + dx1.*dx2.*cos(x2)) + (-dx1.*sin(x3).*cos(x2) + dx2.*cos(x3)).*(-dx4.*sin(x4).*sin(x6) + dx4.*sin(x5).*cos(x4).*cos(x6) + dx5.*sin(x4).*cos(x5).*cos(x6) - dx6.*sin(x4).*sin(x5).*sin(x6) + dx6.*cos(x4).*cos(x6)) + (sin(x4).*sin(x5).*cos(x6) + sin(x6).*cos(x4)).*(-ddx1.*sin(x3).*cos(x2) + ddx2.*cos(x3) + dx1.*dx2.*sin(x2).*sin(x3) - dx1.*dx3.*cos(x2).*cos(x3) - dx2.*dx3.*sin(x3)) + (ddx1.*cos(x2).*cos(x3) + ddx2.*sin(x3) - dx1.*dx2.*sin(x2).*cos(x3) - dx1.*dx3.*sin(x3).*cos(x2) + dx2.*dx3.*cos(x3)).*cos(x5).*cos(x6)) + (-rigid2Cx.*(dx4.*sin(x5) + dx6 + (dx1.*sin(x2) + dx3).*cos(x4).*cos(x5) - (-dx1.*sin(x3).*cos(x2) + dx2.*cos(x3)).*sin(x4).*cos(x5) + (dx1.*cos(x2).*cos(x3) + dx2.*sin(x3)).*sin(x5)) + rigid2Cz.*(dx4.*cos(x5).*cos(x6) + dx5.*sin(x6) + (dx1.*sin(x2) + dx3).*(sin(x4).*sin(x6) - sin(x5).*cos(x4).*cos(x6)) + (-dx1.*sin(x3).*cos(x2) + dx2.*cos(x3)).*(sin(x4).*sin(x5).*cos(x6) + sin(x6).*cos(x4)) + (dx1.*cos(x2).*cos(x3) + dx2.*sin(x3)).*cos(x5).*cos(x6))).*(dx4.*cos(x5).*cos(x6) + dx5.*sin(x6) + (dx1.*sin(x2) + dx3).*(sin(x4).*sin(x6) - sin(x5).*cos(x4).*cos(x6)) + (-dx1.*sin(x3).*cos(x2) + dx2.*cos(x3)).*(sin(x4).*sin(x5).*cos(x6) + sin(x6).*cos(x4)) + (dx1.*cos(x2).*cos(x3) + dx2.*sin(x3)).*cos(x5).*cos(x6)) - (rigid2Cy.*(dx4.*sin(x5) + dx6 + (dx1.*sin(x2) + dx3).*cos(x4).*cos(x5) - (-dx1.*sin(x3).*cos(x2) + dx2.*cos(x3)).*sin(x4).*cos(x5) + (dx1.*cos(x2).*cos(x3) + dx2.*sin(x3)).*sin(x5)) - rigid2Cz.*(-dx4.*sin(x6).*cos(x5) + dx5.*cos(x6) + (dx1.*sin(x2) + dx3).*(sin(x4).*cos(x6) + sin(x5).*sin(x6).*cos(x4)) + (-dx1.*sin(x3).*cos(x2) + dx2.*cos(x3)).*(-sin(x4).*sin(x5).*sin(x6) + cos(x4).*cos(x6)) - (dx1.*cos(x2).*cos(x3) + dx2.*sin(x3)).*sin(x6).*cos(x5))).*(-dx4.*sin(x6).*cos(x5) + dx5.*cos(x6) + (dx1.*sin(x2) + dx3).*(sin(x4).*cos(x6) + sin(x5).*sin(x6).*cos(x4)) + (-dx1.*sin(x3).*cos(x2) + dx2.*cos(x3)).*(-sin(x4).*sin(x5).*sin(x6) + cos(x4).*cos(x6)) - (dx1.*cos(x2).*cos(x3) + dx2.*sin(x3)).*sin(x6).*cos(x5))) + m2.*(-(sin(x1).*sin(x3) - sin(x2).*cos(x1).*cos(x3)).*sin(x6).*cos(x5) + (sin(x1).*cos(x3) + sin(x2).*sin(x3).*cos(x1)).*(-sin(x4).*sin(x5).*sin(x6) + cos(x4).*cos(x6)) + (sin(x4).*cos(x6) + sin(x5).*sin(x6).*cos(x4)).*cos(x1).*cos(x2)).*(-rigid2Cx.*(ddx4.*sin(x5) + ddx6 + dx4.*dx5.*cos(x5) - dx4.*(dx1.*sin(x2) + dx3).*sin(x4).*cos(x5) - dx4.*(-dx1.*sin(x3).*cos(x2) + dx2.*cos(x3)).*cos(x4).*cos(x5) - dx5.*(dx1.*sin(x2) + dx3).*sin(x5).*cos(x4) + dx5.*(-dx1.*sin(x3).*cos(x2) + dx2.*cos(x3)).*sin(x4).*sin(x5) + dx5.*(dx1.*cos(x2).*cos(x3) + dx2.*sin(x3)).*cos(x5) + (ddx1.*sin(x2) + ddx3 + dx1.*dx2.*cos(x2)).*cos(x4).*cos(x5) - (-ddx1.*sin(x3).*cos(x2) + ddx2.*cos(x3) + dx1.*dx2.*sin(x2).*sin(x3) - dx1.*dx3.*cos(x2).*cos(x3) - dx2.*dx3.*sin(x3)).*sin(x4).*cos(x5) + (ddx1.*cos(x2).*cos(x3) + ddx2.*sin(x3) - dx1.*dx2.*sin(x2).*cos(x3) - dx1.*dx3.*sin(x3).*cos(x2) + dx2.*dx3.*cos(x3)).*sin(x5)) + rigid2Cz.*(ddx4.*cos(x5).*cos(x6) + ddx5.*sin(x6) - dx4.*dx5.*sin(x5).*cos(x6) - dx4.*dx6.*sin(x6).*cos(x5) + dx5.*dx6.*cos(x6) - dx5.*(dx1.*cos(x2).*cos(x3) + dx2.*sin(x3)).*sin(x5).*cos(x6) - dx6.*(dx1.*cos(x2).*cos(x3) + dx2.*sin(x3)).*sin(x6).*cos(x5) + (dx1.*sin(x2) + dx3).*(dx4.*sin(x4).*sin(x5).*cos(x6) + dx4.*sin(x6).*cos(x4) - dx5.*cos(x4).*cos(x5).*cos(x6) + dx6.*sin(x4).*cos(x6) + dx6.*sin(x5).*sin(x6).*cos(x4)) + (sin(x4).*sin(x6) - sin(x5).*cos(x4).*cos(x6)).*(ddx1.*sin(x2) + ddx3 + dx1.*dx2.*cos(x2)) + (-dx1.*sin(x3).*cos(x2) + dx2.*cos(x3)).*(-dx4.*sin(x4).*sin(x6) + dx4.*sin(x5).*cos(x4).*cos(x6) + dx5.*sin(x4).*cos(x5).*cos(x6) - dx6.*sin(x4).*sin(x5).*sin(x6) + dx6.*cos(x4).*cos(x6)) + (sin(x4).*sin(x5).*cos(x6) + sin(x6).*cos(x4)).*(-ddx1.*sin(x3).*cos(x2) + ddx2.*cos(x3) + dx1.*dx2.*sin(x2).*sin(x3) - dx1.*dx3.*cos(x2).*cos(x3) - dx2.*dx3.*sin(x3)) + (ddx1.*cos(x2).*cos(x3) + ddx2.*sin(x3) - dx1.*dx2.*sin(x2).*cos(x3) - dx1.*dx3.*sin(x3).*cos(x2) + dx2.*dx3.*cos(x3)).*cos(x5).*cos(x6)) - (rigid2Cx.*(-dx4.*sin(x6).*cos(x5) + dx5.*cos(x6) + (dx1.*sin(x2) + dx3).*(sin(x4).*cos(x6) + sin(x5).*sin(x6).*cos(x4)) + (-dx1.*sin(x3).*cos(x2) + dx2.*cos(x3)).*(-sin(x4).*sin(x5).*sin(x6) + cos(x4).*cos(x6)) - (dx1.*cos(x2).*cos(x3) + dx2.*sin(x3)).*sin(x6).*cos(x5)) - rigid2Cy.*(dx4.*cos(x5).*cos(x6) + dx5.*sin(x6) + (dx1.*sin(x2) + dx3).*(sin(x4).*sin(x6) - sin(x5).*cos(x4).*cos(x6)) + (-dx1.*sin(x3).*cos(x2) + dx2.*cos(x3)).*(sin(x4).*sin(x5).*cos(x6) + sin(x6).*cos(x4)) + (dx1.*cos(x2).*cos(x3) + dx2.*sin(x3)).*cos(x5).*cos(x6))).*(dx4.*cos(x5).*cos(x6) + dx5.*sin(x6) + (dx1.*sin(x2) + dx3).*(sin(x4).*sin(x6) - sin(x5).*cos(x4).*cos(x6)) + (-dx1.*sin(x3).*cos(x2) + dx2.*cos(x3)).*(sin(x4).*sin(x5).*cos(x6) + sin(x6).*cos(x4)) + (dx1.*cos(x2).*cos(x3) + dx2.*sin(x3)).*cos(x5).*cos(x6)) + (rigid2Cy.*(dx4.*sin(x5) + dx6 + (dx1.*sin(x2) + dx3).*cos(x4).*cos(x5) - (-dx1.*sin(x3).*cos(x2) + dx2.*cos(x3)).*sin(x4).*cos(x5) + (dx1.*cos(x2).*cos(x3) + dx2.*sin(x3)).*sin(x5)) - rigid2Cz.*(-dx4.*sin(x6).*cos(x5) + dx5.*cos(x6) + (dx1.*sin(x2) + dx3).*(sin(x4).*cos(x6) + sin(x5).*sin(x6).*cos(x4)) + (-dx1.*sin(x3).*cos(x2) + dx2.*cos(x3)).*(-sin(x4).*sin(x5).*sin(x6) + cos(x4).*cos(x6)) - (dx1.*cos(x2).*cos(x3) + dx2.*sin(x3)).*sin(x6).*cos(x5))).*(dx4.*sin(x5) + dx6 + (dx1.*sin(x2) + dx3).*cos(x4).*cos(x5) - (-dx1.*sin(x3).*cos(x2) + dx2.*cos(x3)).*sin(x4).*cos(x5) + (dx1.*cos(x2).*cos(x3) + dx2.*sin(x3)).*sin(x5))) + m2.*((sin(x1).*sin(x3) - sin(x2).*cos(x1).*cos(x3)).*cos(x5).*cos(x6) + (sin(x1).*cos(x3) + sin(x2).*sin(x3).*cos(x1)).*(sin(x4).*sin(x5).*cos(x6) + sin(x6).*cos(x4)) + (sin(x4).*sin(x6) - sin(x5).*cos(x4).*cos(x6)).*cos(x1).*cos(x2)).*(rigid2Cy.*(ddx4.*sin(x5) + ddx6 + dx4.*dx5.*cos(x5) - dx4.*(dx1.*sin(x2) + dx3).*sin(x4).*cos(x5) - dx4.*(-dx1.*sin(x3).*cos(x2) + dx2.*cos(x3)).*cos(x4).*cos(x5) - dx5.*(dx1.*sin(x2) + dx3).*sin(x5).*cos(x4) + dx5.*(-dx1.*sin(x3).*cos(x2) + dx2.*cos(x3)).*sin(x4).*sin(x5) + dx5.*(dx1.*cos(x2).*cos(x3) + dx2.*sin(x3)).*cos(x5) + (ddx1.*sin(x2) + ddx3 + dx1.*dx2.*cos(x2)).*cos(x4).*cos(x5) - (-ddx1.*sin(x3).*cos(x2) + ddx2.*cos(x3) + dx1.*dx2.*sin(x2).*sin(x3) - dx1.*dx3.*cos(x2).*cos(x3) - dx2.*dx3.*sin(x3)).*sin(x4).*cos(x5) + (ddx1.*cos(x2).*cos(x3) + ddx2.*sin(x3) - dx1.*dx2.*sin(x2).*cos(x3) - dx1.*dx3.*sin(x3).*cos(x2) + dx2.*dx3.*cos(x3)).*sin(x5)) - rigid2Cz.*(-ddx4.*sin(x6).*cos(x5) + ddx5.*cos(x6) + dx4.*dx5.*sin(x5).*sin(x6) - dx4.*dx6.*cos(x5).*cos(x6) - dx5.*dx6.*sin(x6) + dx5.*(dx1.*cos(x2).*cos(x3) + dx2.*sin(x3)).*sin(x5).*sin(x6) - dx6.*(dx1.*cos(x2).*cos(x3) + dx2.*sin(x3)).*cos(x5).*cos(x6) + (dx1.*sin(x2) + dx3).*(-dx4.*sin(x4).*sin(x5).*sin(x6) + dx4.*cos(x4).*cos(x6) + dx5.*sin(x6).*cos(x4).*cos(x5) - dx6.*sin(x4).*sin(x6) + dx6.*sin(x5).*cos(x4).*cos(x6)) + (sin(x4).*cos(x6) + sin(x5).*sin(x6).*cos(x4)).*(ddx1.*sin(x2) + ddx3 + dx1.*dx2.*cos(x2)) + (-dx1.*sin(x3).*cos(x2) + dx2.*cos(x3)).*(-dx4.*sin(x4).*cos(x6) - dx4.*sin(x5).*sin(x6).*cos(x4) - dx5.*sin(x4).*sin(x6).*cos(x5) - dx6.*sin(x4).*sin(x5).*cos(x6) - dx6.*sin(x6).*cos(x4)) + (-sin(x4).*sin(x5).*sin(x6) + cos(x4).*cos(x6)).*(-ddx1.*sin(x3).*cos(x2) + ddx2.*cos(x3) + dx1.*dx2.*sin(x2).*sin(x3) - dx1.*dx3.*cos(x2).*cos(x3) - dx2.*dx3.*sin(x3)) - (ddx1.*cos(x2).*cos(x3) + ddx2.*sin(x3) - dx1.*dx2.*sin(x2).*cos(x3) - dx1.*dx3.*sin(x3).*cos(x2) + dx2.*dx3.*cos(x3)).*sin(x6).*cos(x5)) - (-rigid2Cx.*(dx4.*sin(x5) + dx6 + (dx1.*sin(x2) + dx3).*cos(x4).*cos(x5) - (-dx1.*sin(x3).*cos(x2) + dx2.*cos(x3)).*sin(x4).*cos(x5) + (dx1.*cos(x2).*cos(x3) + dx2.*sin(x3)).*sin(x5)) + rigid2Cz.*(dx4.*cos(x5).*cos(x6) + dx5.*sin(x6) + (dx1.*sin(x2) + dx3).*(sin(x4).*sin(x6) - sin(x5).*cos(x4).*cos(x6)) + (-dx1.*sin(x3).*cos(x2) + dx2.*cos(x3)).*(sin(x4).*sin(x5).*cos(x6) + sin(x6).*cos(x4)) + (dx1.*cos(x2).*cos(x3) + dx2.*sin(x3)).*cos(x5).*cos(x6))).*(dx4.*sin(x5) + dx6 + (dx1.*sin(x2) + dx3).*cos(x4).*cos(x5) - (-dx1.*sin(x3).*cos(x2) + dx2.*cos(x3)).*sin(x4).*cos(x5) + (dx1.*cos(x2).*cos(x3) + dx2.*sin(x3)).*sin(x5)) + (rigid2Cx.*(-dx4.*sin(x6).*cos(x5) + dx5.*cos(x6) + (dx1.*sin(x2) + dx3).*(sin(x4).*cos(x6) + sin(x5).*sin(x6).*cos(x4)) + (-dx1.*sin(x3).*cos(x2) + dx2.*cos(x3)).*(-sin(x4).*sin(x5).*sin(x6) + cos(x4).*cos(x6)) - (dx1.*cos(x2).*cos(x3) + dx2.*sin(x3)).*sin(x6).*cos(x5)) - rigid2Cy.*(dx4.*cos(x5).*cos(x6) + dx5.*sin(x6) + (dx1.*sin(x2) + dx3).*(sin(x4).*sin(x6) - sin(x5).*cos(x4).*cos(x6)) + (-dx1.*sin(x3).*cos(x2) + dx2.*cos(x3)).*(sin(x4).*sin(x5).*cos(x6) + sin(x6).*cos(x4)) + (dx1.*cos(x2).*cos(x3) + dx2.*sin(x3)).*cos(x5).*cos(x6))).*(-dx4.*sin(x6).*cos(x5) + dx5.*cos(x6) + (dx1.*sin(x2) + dx3).*(sin(x4).*cos(x6) + sin(x5).*sin(x6).*cos(x4)) + (-dx1.*sin(x3).*cos(x2) + dx2.*cos(x3)).*(-sin(x4).*sin(x5).*sin(x6) + cos(x4).*cos(x6)) - (dx1.*cos(x2).*cos(x3) + dx2.*sin(x3)).*sin(x6).*cos(x5))) + (m1.*(-rigid1Cx.*(ddx1.*sin(x2) + ddx3 + dx1.*dx2.*cos(x2)) + rigid1Cz.*(ddx1.*cos(x2).*cos(x3) + ddx2.*sin(x3) - dx1.*dx2.*sin(x2).*cos(x3) - dx1.*dx3.*sin(x3).*cos(x2) + dx2.*dx3.*cos(x3)) + (dx1.*sin(x2) + dx3).*(rigid1Cy.*(dx1.*sin(x2) + dx3) - rigid1Cz.*(-dx1.*sin(x3).*cos(x2) + dx2.*cos(x3))) - (rigid1Cx.*(-dx1.*sin(x3).*cos(x2) + dx2.*cos(x3)) - rigid1Cy.*(dx1.*cos(x2).*cos(x3) + dx2.*sin(x3))).*(dx1.*cos(x2).*cos(x3) + dx2.*sin(x3))) + m2.*(-rigid1Cx.*(ddx1.*sin(x2) + ddx3 + dx1.*dx2.*cos(x2)) + rigid1Cz.*(ddx1.*cos(x2).*cos(x3) + ddx2.*sin(x3) - dx1.*dx2.*sin(x2).*cos(x3) - dx1.*dx3.*sin(x3).*cos(x2) + dx2.*dx3.*cos(x3)) + rigid1Px.*(ddx1.*sin(x2) + ddx3 + dx1.*dx2.*cos(x2)) - rigid1Pz.*(ddx1.*cos(x2).*cos(x3) + ddx2.*sin(x3) - dx1.*dx2.*sin(x2).*cos(x3) - dx1.*dx3.*sin(x3).*cos(x2) + dx2.*dx3.*cos(x3)) + (dx1.*sin(x2) + dx3).*(rigid1Cy.*(dx1.*sin(x2) + dx3) - rigid1Cz.*(-dx1.*sin(x3).*cos(x2) + dx2.*cos(x3)) - rigid1Py.*(dx1.*sin(x2) + dx3) + rigid1Pz.*(-dx1.*sin(x3).*cos(x2) + dx2.*cos(x3))) - (dx1.*cos(x2).*cos(x3) + dx2.*sin(x3)).*(rigid1Cx.*(-dx1.*sin(x3).*cos(x2) + dx2.*cos(x3)) - rigid1Cy.*(dx1.*cos(x2).*cos(x3) + dx2.*sin(x3)) - rigid1Px.*(-dx1.*sin(x3).*cos(x2) + dx2.*cos(x3)) + rigid1Py.*(dx1.*cos(x2).*cos(x3) + dx2.*sin(x3))))).*(sin(x1).*cos(x3) + sin(x2).*sin(x3).*cos(x1)) + (m1.*(rigid1Cx.*(-ddx1.*sin(x3).*cos(x2) + ddx2.*cos(x3) + dx1.*dx2.*sin(x2).*sin(x3) - dx1.*dx3.*cos(x2).*cos(x3) - dx2.*dx3.*sin(x3)) - rigid1Cy.*(ddx1.*cos(x2).*cos(x3) + ddx2.*sin(x3) - dx1.*dx2.*sin(x2).*cos(x3) - dx1.*dx3.*sin(x3).*cos(x2) + dx2.*dx3.*cos(x3)) + (-rigid1Cx.*(dx1.*sin(x2) + dx3) + rigid1Cz.*(dx1.*cos(x2).*cos(x3) + dx2.*sin(x3))).*(dx1.*cos(x2).*cos(x3) + dx2.*sin(x3)) - (rigid1Cy.*(dx1.*sin(x2) + dx3) - rigid1Cz.*(-dx1.*sin(x3).*cos(x2) + dx2.*cos(x3))).*(-dx1.*sin(x3).*cos(x2) + dx2.*cos(x3))) + m2.*(rigid1Cx.*(-ddx1.*sin(x3).*cos(x2) + ddx2.*cos(x3) + dx1.*dx2.*sin(x2).*sin(x3) - dx1.*dx3.*cos(x2).*cos(x3) - dx2.*dx3.*sin(x3)) - rigid1Cy.*(ddx1.*cos(x2).*cos(x3) + ddx2.*sin(x3) - dx1.*dx2.*sin(x2).*cos(x3) - dx1.*dx3.*sin(x3).*cos(x2) + dx2.*dx3.*cos(x3)) - rigid1Px.*(-ddx1.*sin(x3).*cos(x2) + ddx2.*cos(x3) + dx1.*dx2.*sin(x2).*sin(x3) - dx1.*dx3.*cos(x2).*cos(x3) - dx2.*dx3.*sin(x3)) + rigid1Py.*(ddx1.*cos(x2).*cos(x3) + ddx2.*sin(x3) - dx1.*dx2.*sin(x2).*cos(x3) - dx1.*dx3.*sin(x3).*cos(x2) + dx2.*dx3.*cos(x3)) - (-dx1.*sin(x3).*cos(x2) + dx2.*cos(x3)).*(rigid1Cy.*(dx1.*sin(x2) + dx3) - rigid1Cz.*(-dx1.*sin(x3).*cos(x2) + dx2.*cos(x3)) - rigid1Py.*(dx1.*sin(x2) + dx3) + rigid1Pz.*(-dx1.*sin(x3).*cos(x2) + dx2.*cos(x3))) + (dx1.*cos(x2).*cos(x3) + dx2.*sin(x3)).*(-rigid1Cx.*(dx1.*sin(x2) + dx3) + rigid1Cz.*(dx1.*cos(x2).*cos(x3) + dx2.*sin(x3)) + rigid1Px.*(dx1.*sin(x2) + dx3) - rigid1Pz.*(dx1.*cos(x2).*cos(x3) + dx2.*sin(x3))))).*cos(x1).*cos(x2) + (m1.*(rigid1Cy.*(ddx1.*sin(x2) + ddx3 + dx1.*dx2.*cos(x2)) - rigid1Cz.*(-ddx1.*sin(x3).*cos(x2) + ddx2.*cos(x3) + dx1.*dx2.*sin(x2).*sin(x3) - dx1.*dx3.*cos(x2).*cos(x3) - dx2.*dx3.*sin(x3)) - (dx1.*sin(x2) + dx3).*(-rigid1Cx.*(dx1.*sin(x2) + dx3) + rigid1Cz.*(dx1.*cos(x2).*cos(x3) + dx2.*sin(x3))) + (rigid1Cx.*(-dx1.*sin(x3).*cos(x2) + dx2.*cos(x3)) - rigid1Cy.*(dx1.*cos(x2).*cos(x3) + dx2.*sin(x3))).*(-dx1.*sin(x3).*cos(x2) + dx2.*cos(x3))) + m2.*(rigid1Cy.*(ddx1.*sin(x2) + ddx3 + dx1.*dx2.*cos(x2)) - rigid1Cz.*(-ddx1.*sin(x3).*cos(x2) + ddx2.*cos(x3) + dx1.*dx2.*sin(x2).*sin(x3) - dx1.*dx3.*cos(x2).*cos(x3) - dx2.*dx3.*sin(x3)) - rigid1Py.*(ddx1.*sin(x2) + ddx3 + dx1.*dx2.*cos(x2)) + rigid1Pz.*(-ddx1.*sin(x3).*cos(x2) + ddx2.*cos(x3) + dx1.*dx2.*sin(x2).*sin(x3) - dx1.*dx3.*cos(x2).*cos(x3) - dx2.*dx3.*sin(x3)) - (dx1.*sin(x2) + dx3).*(-rigid1Cx.*(dx1.*sin(x2) + dx3) + rigid1Cz.*(dx1.*cos(x2).*cos(x3) + dx2.*sin(x3)) + rigid1Px.*(dx1.*sin(x2) + dx3) - rigid1Pz.*(dx1.*cos(x2).*cos(x3) + dx2.*sin(x3))) + (-dx1.*sin(x3).*cos(x2) + dx2.*cos(x3)).*(rigid1Cx.*(-dx1.*sin(x3).*cos(x2) + dx2.*cos(x3)) - rigid1Cy.*(dx1.*cos(x2).*cos(x3) + dx2.*sin(x3)) - rigid1Px.*(-dx1.*sin(x3).*cos(x2) + dx2.*cos(x3)) + rigid1Py.*(dx1.*cos(x2).*cos(x3) + dx2.*sin(x3))))).*(sin(x1).*sin(x3) - sin(x2).*cos(x1).*cos(x3))];

== matlab function double_3D_pend/MATLAB Function3 ==
  data: u input; Izz parameter; Iyy parameter; Ixx parameter; g parameter; l parameter; m parameter; y output; q1new output; q2new output; akt input; l0m parameter; force parameter; u1 output
function [y,q1new,q2new,u1]  = fcn(u,Izz, Iyy, Ixx, g, l, m,akt, l0m, force)
t = 0;

y = zeros(16,1);
q1 = [u(7);u(1:3)];
q2 = [u(8);u(4:6)];
q1new = q1/norm(q1);
q2new = q2/norm(q2);
qnew = [q1new(2:4);q2new(2:4);q1new(1);q2new(1)];
u1 = u(9:11);

FM = FE_Q(0,[q1new;q2new]',force,l0m,akt');
% MM = mm(t,[q1new;q2new]',u(9:end)',Ixx,Iyy,Izz,l,m, g);
% FE = fe(t,[q1new;q2new]',u(9:end)',Ixx,Iyy,Izz,l,m, g);

MM = mm(t,qnew',u(9:end)',Ixx,Iyy,Izz,l,m, g);
FE = fe(t,qnew',u(9:end)',Ixx,Iyy,Izz,l,m, g);
y = MM\(FE+[zeros(8,1);FM;0;0]); %

function res = G(Q)
Q0 = Q(1);
Q1 = Q(2);
Q2 = Q(3);
Q3 = Q(4);
res = [-Q1, Q0, Q3, -Q2;
        -Q2,-Q3, Q0, Q1;
        -Q3, Q2, -Q1, Q0];
end
end

== matlab function double_3D_pend/MATLAB Function4 ==
  data: u input; y output; q input; qd input
function y = fcn(u,q,qd)

y = 1/2*G(q)'*u - qd;

function res = G(Q)
Q0 = Q(1);
Q1 = Q(2);
Q2 = Q(3);
Q3 = Q(4);
res = [-Q1, Q0, Q3, -Q2;
        -Q2,-Q3, Q0, Q1;
        -Q3, Q2, -Q1, Q0];
end
end

== matlab function double_3D_pend/DELT1/Passive_force_norm ==
  data: lm input; Fp_norm output; l0 input
function Fp_norm = fcn(lm,l0)
Fp_norm = ((lm/l0)^3)*exp(8*lm/l0-12.9);

== matlab function double_3D_pend/DELT2/Active_factor_norm ==
  data: Fa_norm output; lm input; l0 input; a input
function Fa_norm = fcn(lm,l0,a)
f_gauss = 0.25;
Fa_norm = (exp(-(lm/l0-1)^2/f_gauss))*a;

== matlab function double_3D_pend/DELT2/Passive_force_norm ==
  data: lm input; Fp_norm output; l0 input
function Fp_norm = fcn(lm,l0)
Fp_norm = ((lm/l0)^3)*exp(8*lm/l0-12.9);

== matlab function double_3D_pend/DELT3/Active_factor_norm ==
  data: Fa_norm output; lm input; l0 input; a input
function Fa_norm = fcn(lm,l0,a)
f_gauss = 0.25;
Fa_norm = (exp(-(lm/l0-1)^2/f_gauss))*a;

== matlab function double_3D_pend/DELT3/Passive_force_norm ==
  data: lm input; Fp_norm output; l0 input
function Fp_norm = fcn(lm,l0)
Fp_norm = ((lm/l0)^3)*exp(8*lm/l0-12.9);

== matlab function double_3D_pend/MATLAB Function ==
  data: t input; x input; IU parameter; IL parameter; m parameter; c parameter; k parameter; y output; g parameter; rigid1C parameter; rigid1P parameter; rigid2C parameter; force parameter; l0m parameter; akt input
function y = fcn(t,x,IU,IL,m,c,k,g,rigid1C, rigid1P, rigid2C,force, l0m, akt)
%, sh_e, T_el, eps, k_contact, cont_P, akt, force, l0m
IU = [IU(1:3),IU(6),IU(4),IU(5)];
IL = [IL(1:3),IL(6),IL(4),IL(5)];
y = zeros(12,1);
MM = mm(t,x(1:6)',IU,IL,m,c,k,g,rigid1C,rigid1P,rigid2C);
FO = fo(t,x',IU,IL,m,c,k,g,rigid1C,rigid1P,rigid2C);
FE = fe(t,[x(1:6)',x(7:12)'],force,l0m,akt');
y = MM\(FO+FE);
